simulink library "Ampere_Library"  (R2022b)
settings: Solver=FixedStepDiscrete  StartTime=0  StopTime=10.0  RelTol=1e-3  EnableMultiTasking=on
undefined symbols (not defined in the file or in its folder): A_INST_double, Dem_EventStatusType, ECU_AMBIENT_TEMPERATURE, SET_ECU_AMBIENT_TEMPERATURE, SlDemoSign, Std_ReturnType
libraries: simulink x13
(part 9 of 10)

== system Ampere_Library/User_Defined_Libraries/Timers_and_Counters/A_COUNTER ==
  note: Refer Mask Description of this Library block for detailed information.
  start_flag : Inport  OutDataTypeStr=boolean
      settings: AttributesFormatString=DT = %<OutDataTypeStr>
  ClrVal : Constant  Value=ClrVal  OutDataTypeStr=Inherit: Inherit via back propagation
  IncrVal : Constant  Value=IncrVal  OutDataTypeStr=Inherit: Inherit via back propagation
  Min : MinMax  Inputs=2  InputSameDT=on  RndMeth=Zero
      settings: AttributesFormatString=SAT = %<SaturateOnIntegerOverflow>
  Sum1 : Sum  InputSameDT=on  RndMeth=Zero
      settings: AttributesFormatString=SAT = %<SaturateOnIntegerOverflow>
  Switch1 : Switch  Criteria=u2 ~= 0  Threshold=0.5  RndMeth=Zero  SaturateOnIntegerOverflow=off
      settings: AttributesFormatString=SAT = %<SaturateOnIntegerOverflow>
  UnitDelay : UnitDelay  InitialCondition=IC_zero  SampleTime=-1  HasFrameUpgradeWarning=on
      settings: AttributesFormatString=Init = %<InitialCondition>
  limit_value : Constant  Value=limit_value
  count_value : Outport
  wires:
  start_flag/1 -> Switch1/2
  Sum1/1 -> Min/2
  ClrVal/1 -> Switch1/3
  Switch1/1 -> UnitDelay/1, count_value/1
  IncrVal/1 -> Sum1/2
  Min/1 -> Switch1/1
  limit_value/1 -> Min/1
  UnitDelay/1 -> Sum1/1

== system Ampere_Library/User_Defined_Libraries/Timers_and_Counters/A_Counter_Hold ==
  note: Refer Mask Description of this Library block for detailed information.
  start_flag : Inport  OutDataTypeStr=boolean
      settings: AttributesFormatString=DT = %<OutDataTypeStr>
  clear_flag : Inport  Port=2  OutDataTypeStr=boolean
      settings: AttributesFormatString=DT = %<OutDataTypeStr>
  ClrVal : Constant  Value=ClrVal  OutDataTypeStr=Inherit: Inherit via back propagation
  HoldVal : Constant  Value=HoldVal  OutDataTypeStr=Inherit: Inherit via back propagation
  MinMax : MinMax  Inputs=2  InputSameDT=on  RndMeth=Zero  SaturateOnIntegerOverflow=on
      settings: AttributesFormatString=SAT= %<SaturateOnIntegerOverflow>
  SetVal : Constant  Value=SetVal  OutDataTypeStr=Inherit: Inherit via back propagation
  Sum1 : Sum  InputSameDT=on  RndMeth=Zero  SaturateOnIntegerOverflow=on
      settings: AttributesFormatString=SAT = %<SaturateOnIntegerOverflow>
  Switch : Switch  Criteria=u2 ~= 0  Threshold=0.5  RndMeth=Zero
      settings: AttributesFormatString=SAT = %<SaturateOnIntegerOverflow>
  Switch1 : Switch  Criteria=u2 ~= 0  Threshold=0.5  RndMeth=Zero
      settings: AttributesFormatString=SAT = %<SaturateOnIntegerOverflow>
  UnitDelay : UnitDelay  InitialCondition=count_hold_init  SampleTime=-1  HasFrameUpgradeWarning=on
      settings: AttributesFormatString=Init = %<InitialCondition>\n
  limit_value : Constant  Value=limit_value
  count_value : Outport
  wires:
  SetVal/1 -> Switch/1
  Switch/1 -> Sum1/1
  Sum1/1 -> MinMax/2
  start_flag/1 -> Switch/2
  clear_flag/1 -> Switch1/2
  Switch1/1 -> UnitDelay/1, count_value/1
  HoldVal/1 -> Switch/3
  limit_value/1 -> MinMax/1
  UnitDelay/1 -> Sum1/2
  MinMax/1 -> Switch1/3
  ClrVal/1 -> Switch1/1

== system Ampere_Library/User_Defined_Libraries/Timers_and_Counters/A_IncAndDecCounter ==
  note: Refer Mask Description of this Library block for detailed information.
  Inc_Counter : Inport  OutDataTypeStr=boolean
      settings: AttributesFormatString=DT = %<OutDataTypeStr>
  Dec_Counter : Inport  Port=2  OutDataTypeStr=boolean
      settings: AttributesFormatString=DT = %<OutDataTypeStr>
  Max_Counter : Inport  Port=3
  Min_Counter : Inport  Port=4
  Reset_Counter : Inport  Port=5  OutDataTypeStr=boolean
      settings: AttributesFormatString=DT = %<OutDataTypeStr>
  Counter_Step : Inport  Port=6
  Init_Counter : Inport  Port=7
  Add1 : Sum  InputSameDT=on  RndMeth=Zero
      settings: AttributesFormatString=SAT = %<SaturateOnIntegerOverflow>\n
  Add2 : Sum  Inputs=+-  InputSameDT=on  RndMeth=Zero
      settings: AttributesFormatString=SAT = %<SaturateOnIntegerOverflow>\n
  CONS_ONE : Constant  Value=Cons_One
  CONS_THREE : Constant  Value=Cons_Three
  CONS_TWO : Constant  Value=Cons_Two
  CONS_ZERO : Constant  Value=Cons_Zero
  CONS_ZERO_BP : Constant  Value=Cons_Zero_BP  OutDataTypeStr=Inherit: Inherit via back propagation
  MinMax : MinMax  Inputs=2  InputSameDT=on  RndMeth=Zero
      settings: AttributesFormatString=SAT = %<SaturateOnIntegerOverflow>
  MinMax1 : MinMax  Function=max  Inputs=2  InputSameDT=on  RndMeth=Zero
      settings: AttributesFormatString=SAT = %<SaturateOnIntegerOverflow>
  Multiport_Switch : MultiPortSwitch  DataPortOrder=Zero-based contiguous  DataPortForDefault=Additional data port  DiagnosticForDefault=None  zeroidx=on  RndMeth=Zero  SaturateOnIntegerOverflow=off
      settings: AttributesFormatString=SAT = %<SaturateOnIntegerOverflow>
  Switch{,2..4} (4 alike) : Switch  Criteria=u2 ~= 0  RndMeth=Zero  SaturateOnIntegerOverflow=off
      Switch settings: AttributesFormatString=SAT = %<SaturateOnIntegerOverflow>
  UnitDelay : UnitDelay  InitialCondition=true  SampleTime=-1  HasFrameUpgradeWarning=on
      settings: AttributesFormatString=Init = %<InitialCondition>\n
  Unit_Delay1 : UnitDelay  InitialCondition=false  SampleTime=-1  HasFrameUpgradeWarning=on
      settings: AttributesFormatString=Init = %<InitialCondition>\n
  false : Constant  Value=false
  Counter_Out : Outport
  wires:
  Counter_Step/1 -> Add2/2, Add1/1
  UnitDelay/1 -> Switch/2
  Init_Counter/1 -> Switch/1
  Multiport_Switch/1 -> MinMax/1
  CONS_THREE/1 -> Switch3/3
  MinMax1/1 -> Switch/3
  Min_Counter/1 -> MinMax1/2
  Switch/1 -> Counter_Out/1, Unit_Delay1/1
  CONS_ZERO/1 -> Switch4/1
  MinMax/1 -> MinMax1/1
  Switch2/1 -> Switch4/3
  Unit_Delay1/1 -> Multiport_Switch/5, Add2/1, Add1/2
  Dec_Counter/1 -> Switch2/2
  CONS_ONE/1 -> Switch2/1
  Add2/1 -> Multiport_Switch/3
  Add1/1 -> Multiport_Switch/2
  CONS_TWO/1 -> Switch3/1
  false/1 -> UnitDelay/1
  Switch3/1 -> Switch2/3
  CONS_ZERO_BP/1 -> Multiport_Switch/4
  Switch4/1 -> Multiport_Switch/1
  Max_Counter/1 -> MinMax/2
  Reset_Counter/1 -> Switch3/2
  Inc_Counter/1 -> Switch4/2

== system Ampere_Library/User_Defined_Libraries/Timers_and_Counters/A_Timer_Conversion ==
  note: Refer Mask Description of this Library block for detailed information.
  Timer_To_Adapt : Inport
  Divide : Product  Inputs=*/  RndMeth=Zero
      settings: AttributesFormatString=SAT = %<SaturateOnIntegerOverflow>\n
  RelationalOperator1 : RelationalOperator  Operator=>  OutDataTypeStr=boolean  RndMeth=Zero
  SAMPLE_TIME_CST : Constant  Value=SampleTimeCst  OutDataTypeStr=Inherit: Inherit via back propagation
  Switch : Switch  Criteria=u2 ~= 0  RndMeth=Zero  SaturateOnIntegerOverflow=off
      settings: AttributesFormatString=SAT = %<SaturateOnIntegerOverflow>
  ZERO_CST : Constant  Value=Cons_0  OutDataTypeStr=uint8
      settings: AttributesFormatString=DT = %<OutDataTypeStr>\n
  Timer_Adapted : Outport
  wires:
  Divide/1 -> Switch/1
  Switch/1 -> Timer_Adapted/1
  Timer_To_Adapt/1 -> Divide/1, Switch/3
  RelationalOperator1/1 -> Switch/2
  SAMPLE_TIME_CST/1 -> Divide/2, RelationalOperator1/1
  ZERO_CST/1 -> RelationalOperator1/2

== system Ampere_Library/User_Defined_Libraries/Timers_and_Counters/A_Timer_Dec_Order ==
  note: Detect Increase
  note: Refer Mask Description of this Library block for detailed information.
  Init : Inport
  Duration : Inport  Port=2
  Constant : Constant  Value=Boosting_Factor  OutDataTypeStr=Constant_DT
      settings: AttributesFormatString=DT = %<OutDataTypeStr>\n
  Constant1 : Constant  Value=Boosting_Factor  OutDataTypeStr=Constant_DT
      settings: AttributesFormatString=DT = %<OutDataTypeStr>\n
  Constant2 : Constant  Value=Boosting_Factor  OutDataTypeStr=Constant_DT
      settings: AttributesFormatString=DT = %<OutDataTypeStr>\n
  DataTypeDuplicate : DataTypeDuplicate
  DelayInput1 : UnitDelay  Description=\nStore in Global RAM  InitialCondition=timeoutinit  SampleTime=-1  HasFrameUpgradeWarning=on
      settings: AttributesFormatString=Init = %<InitialCondition>
  DelayInput2 : UnitDelay  Description=\nStore in Global RAM  InitialCondition=Tim1Ini  SampleTime=-1  HasFrameUpgradeWarning=on
      settings: AttributesFormatString=Init = %<InitialCondition>
  DelayInput3 : UnitDelay  Description=\nStore in Global RAM  InitialCondition=initinit  SampleTime=-1  HasFrameUpgradeWarning=on
      settings: AttributesFormatString=Init = %<InitialCondition>
  LogicalOperator : Logic  OutDataTypeStr=boolean
  LogicalOperator1 : Logic  OutDataTypeStr=boolean
  LogicalOperator3 : Logic  Operator=NOT  Inputs=1  OutDataTypeStr=boolean
  Product2 : Product  Inputs=*/  OutDataTypeStr=single  RndMeth=Zero
      settings: AttributesFormatString=DT = %<OutDataTypeStr>\nSAT = %<SaturateOnIntegerOverflow>
  Product3 : Product  OutDataTypeStr=Inherit: Inherit via back propagation  RndMeth=Zero
      settings: AttributesFormatString=SAT = %<SaturateOnIntegerOverflow>
  Product4 : Product  OutDataTypeStr=Inherit: Inherit via back propagation  RndMeth=Zero
      settings: AttributesFormatString=SAT = %<SaturateOnIntegerOverflow>
  RelationalOperator1 : RelationalOperator  Operator=>  OutDataTypeStr=boolean  ZeroCross=off  RndMeth=Zero
  RelationalOperator2 : RelationalOperator  Operator=<=  OutDataTypeStr=boolean  ZeroCross=off  RndMeth=Zero
  Sum : Sum  Inputs=+-  InputSameDT=on  RndMeth=Zero
      settings: AttributesFormatString=SAT = %<SaturateOnIntegerOverflow>
  Switch{1..4} (4 alike) : Switch  Criteria=u2 ~= 0  RndMeth=Zero  SaturateOnIntegerOverflow=off
      Switch2 settings: AttributesFormatString=SAT = %<SaturateOnIntegerOverflow>
      Switch3 settings: AttributesFormatString=SAT = %<SaturateOnIntegerOverflow>
      Switch4 settings: AttributesFormatString=SAT = %<SaturateOnIntegerOverflow>
  TIM1INI3 : Constant  Value=Tim1Ini  OutDataTypeStr=Inherit: Inherit via back propagation
  st : Constant  Value=st  OutDataTypeStr=SampleDT
      settings: AttributesFormatString=DT = %<OutDataTypeStr>\n
  Timeout : Outport
  Timer : Outport  Port=2
  wires:
  Switch3/1 -> Product2/1, DelayInput2/1
  LogicalOperator3/1 -> LogicalOperator1/2
  Duration/1 -> DataTypeDuplicate/2, Product4/1
  Product2/1 -> Timer/1
  Sum/1 -> Switch4/1
  RelationalOperator2/1 -> Switch4/2
  [dly] -> Switch2/1
  Product4/1 -> [dly]
  [Timestep1] -> RelationalOperator1/1
  [Tim1Ini] -> Switch3/1
  DelayInput1/1 -> Switch1/3
  Switch2/1 -> Switch3/3, RelationalOperator1/2
  Init/1 -> LogicalOperator1/1, DelayInput3/1
  Switch1/1 -> LogicalOperator/1, DelayInput1/1
  Product3/1 -> Sum/2, RelationalOperator2/1, [Timestep1]
  Constant1/1 -> Product2/2
  LogicalOperator1/1 -> Switch1/1, Switch1/2, Switch2/2
  LogicalOperator/1 -> Timeout/1
  DelayInput3/1 -> LogicalOperator3/1
  DelayInput2/1 -> RelationalOperator2/2, Sum/1
  Constant/1 -> Product4/2
  st/1 -> Product3/1
  TIM1INI3/1 -> DataTypeDuplicate/1, Switch4/3, [Tim1Ini]
  RelationalOperator1/1 -> Switch3/2, LogicalOperator/2
  Switch4/1 -> Switch2/3
  Constant2/1 -> Product3/2

== system Ampere_Library/User_Defined_Libraries/Timers_and_Counters/A_Timer_Ext_TimeSt ==
  note: Detect Increase
  note: Refer Mask Description of this Library block for detailed information.
  Init : Inport
  Duration : Inport  Port=2
  Timestep : Inport  Port=3
  BOOSTING_FLP : Constant  Value=Boosting_FLP  OutDataTypeStr=Constant_DT
      settings: AttributesFormatString=DT = %<OutDataTypeStr>\n
  BOOSTING_FLP1 : Constant  Value=Boosting_FLP  OutDataTypeStr=Constant_DT
      settings: AttributesFormatString=DT = %<OutDataTypeStr>\n
  BOOSTING_FLP2 : Constant  Value=Boosting_FLP  OutDataTypeStr=Constant_DT
      settings: AttributesFormatString=DT = %<OutDataTypeStr>\n
  DataTypeDuplicate : DataTypeDuplicate  NumInputPorts=3
  DelayInput1 : UnitDelay  Description=\nStore in Global RAM  InitialCondition=timeoutinit  SampleTime=-1  HasFrameUpgradeWarning=on
      settings: AttributesFormatString=Init = %<InitialCondition>\n
  DelayInput2 : UnitDelay  Description=\nStore in Global RAM  InitialCondition=Tim1Ini  SampleTime=-1  HasFrameUpgradeWarning=on
      settings: AttributesFormatString=Init = %<InitialCondition>\n
  DelayInput3 : UnitDelay  Description=\nStore in Global RAM  InitialCondition=initinit  SampleTime=-1  HasFrameUpgradeWarning=on
      settings: AttributesFormatString=Init = %<InitialCondition>\n
  LogicalOperator : Logic  OutDataTypeStr=boolean
  LogicalOperator1 : Logic  OutDataTypeStr=boolean
  LogicalOperator3 : Logic  Operator=NOT  Inputs=1  OutDataTypeStr=boolean
  Product : Product  OutDataTypeStr=Inherit: Inherit via back propagation  RndMeth=Zero
      settings: AttributesFormatString=SAT = %<SaturateOnIntegerOverflow>
  Product1 : Product  OutDataTypeStr=Inherit: Inherit via back propagation  RndMeth=Zero
      settings: AttributesFormatString=SAT = %<SaturateOnIntegerOverflow>
  Product2 : Product  Inputs=*/  OutDataTypeStr=Inherit: Inherit via back propagation  RndMeth=Zero
      settings: AttributesFormatString=SAT = %<SaturateOnIntegerOverflow>
  RelationalOperator1 : RelationalOperator  Operator=>  OutDataTypeStr=boolean  ZeroCross=off  RndMeth=Zero
  RelationalOperator2 : RelationalOperator  Operator=<=  OutDataTypeStr=boolean  ZeroCross=off  RndMeth=Zero
  Sum : Sum  Inputs=+-  InputSameDT=on  RndMeth=Zero
      settings: AttributesFormatString=SAT = %<SaturateOnIntegerOverflow>
  Switch{1..4} (4 alike) : Switch  Criteria=u2 ~= 0  RndMeth=Zero  SaturateOnIntegerOverflow=off
      Switch2 settings: AttributesFormatString=SAT = %<SaturateOnIntegerOverflow>
      Switch3 settings: AttributesFormatString=SAT = %<SaturateOnIntegerOverflow>
      Switch4 settings: AttributesFormatString=SAT = %<SaturateOnIntegerOverflow>
  TIM1INI1 : Constant  Value=Tim1Ini  OutDataTypeStr=Inherit: Inherit via back propagation
  Timeout : Outport
  Timer : Outport  Port=2
  wires:
  DelayInput2/1 -> RelationalOperator2/2, Sum/1
  LogicalOperator1/1 -> Switch1/2, Switch1/1, Switch2/2
  Timestep/1 -> Product/1, DataTypeDuplicate/2
  [Tim1Ini] -> Switch4/3
  [Timestep1] -> RelationalOperator1/1
  [Tim1Ini] -> Switch3/1
  Init/1 -> DelayInput3/1, LogicalOperator1/1
  Switch3/1 -> Product2/1, DelayInput2/1
  LogicalOperator3/1 -> LogicalOperator1/2
  LogicalOperator/1 -> Timeout/1
  Switch1/1 -> DelayInput1/1, LogicalOperator/1
  DelayInput3/1 -> LogicalOperator3/1
  DelayInput1/1 -> Switch1/3
  Switch2/1 -> RelationalOperator1/2, Switch3/3
  Duration/1 -> Product1/1, DataTypeDuplicate/1
  RelationalOperator2/1 -> Switch4/2
  RelationalOperator1/1 -> Switch3/2, LogicalOperator/2
  Switch4/1 -> Switch2/3
  TIM1INI1/1 -> DataTypeDuplicate/3, [Tim1Ini]
  Sum/1 -> Switch4/1
  BOOSTING_FLP1/1 -> Product1/2
  Product2/1 -> Timer/1
  BOOSTING_FLP2/1 -> Product2/2
  Product1/1 -> Switch2/1
  Product/1 -> [Timestep1], RelationalOperator2/1, Sum/2
  BOOSTING_FLP/1 -> Product/2

== system Ampere_Library/User_Defined_Libraries/Timers_and_Counters/A_Timer_Hold_Inc_Order ==
  note: Refer Mask Description of this Library block for detailed information.
  start_flag : Inport
  clear_flag : Inport  Port=2
  target_time : Inport  Port=3
  ClrVal : Constant  Value=ClrVal  OutDataTypeStr=Inherit: Inherit via back propagation
  LogicalOperator2 : Logic  Operator=OR  OutDataTypeStr=boolean
  LogicalOperator3 : Logic  OutDataTypeStr=boolean
  LogicalOperator4 : Logic  Operator=NOT  OutDataTypeStr=boolean
  LogicalOperator5 : Logic  OutDataTypeStr=boolean
  LogicalOperator6 : Logic  Operator=NOT  OutDataTypeStr=boolean
  LogicalOperator7 : Logic  Operator=OR  OutDataTypeStr=boolean
  LogicalOperator8 : Logic  OutDataTypeStr=boolean
  MinMax : MinMax  Inputs=2  InputSameDT=on  RndMeth=Zero
  RelationalOperator : RelationalOperator  Operator=<=  OutDataTypeStr=boolean  RndMeth=Zero
  RelationalOperator1 : RelationalOperator  Operator=<=  OutDataTypeStr=boolean  RndMeth=Zero
  Resol : Constant  Value=Resol  OutDataTypeStr=Inherit: Inherit via back propagation
  Sum : Sum  InputSameDT=on  RndMeth=Zero
  Sum1 : Sum  InputSameDT=on  RndMeth=Zero
  Switch{,1..3} (4 alike) : Switch  Criteria=u2 ~= 0  Threshold=0.5  RndMeth=Zero  SaturateOnIntegerOverflow=off
  TimKill : Constant  Value=TimKill  OutDataTypeStr=Inherit: Inherit via back propagation
  UnitDelay : UnitDelay  InitialCondition=sample_time_init  SampleTime=-1  HasFrameUpgradeWarning=on
      settings: AttributesFormatString=Init = %<InitialCondition>\n
  UnitDelay1 : UnitDelay  InitialCondition=false  SampleTime=-1  HasFrameUpgradeWarning=on
      settings: AttributesFormatString=Init = %<InitialCondition>\n
  UnitDelay2 : UnitDelay  InitialCondition=alarm_init  SampleTime=-1  HasFrameUpgradeWarning=on
      settings: AttributesFormatString=Init = %<InitialCondition>\n
  sample_time : Constant  Value=SampleTime  OutDataTypeStr=Inherit: Inherit via back propagation
  alarm : Outport
  timer_value : Outport  Port=2
  wires:
  LogicalOperator3/1 -> Switch1/1, LogicalOperator5/1, UnitDelay1/1
  Switch1/1 -> alarm/1
  Sum/1 -> Switch/1
  RelationalOperator/1 -> Switch1/3
  LogicalOperator2/1 -> LogicalOperator3/2
  LogicalOperator6/1 -> LogicalOperator3/1, LogicalOperator8/1
  clear_flag/1 -> LogicalOperator7/2, LogicalOperator6/1
  sample_time/1 -> Sum/1
  UnitDelay/1 -> Sum/2, Switch/3
  start_flag/1 -> Switch/2, LogicalOperator8/2
  Switch2/1 -> MinMax/2
  LogicalOperator4/1 -> LogicalOperator5/2
  LogicalOperator8/1 -> LogicalOperator2/1
  LogicalOperator7/1 -> Switch2/2
  UnitDelay1/1 -> LogicalOperator2/2, LogicalOperator4/1
  MinMax/1 -> UnitDelay/1, timer_value/1, Sum1/2
  target_time/1 -> Switch3/1
  TimKill/1 -> RelationalOperator1/2
  Switch3/1 -> RelationalOperator1/1, RelationalOperator/1, UnitDelay2/1, MinMax/1
  ClrVal/1 -> Switch2/1
  RelationalOperator1/1 -> Switch1/2
  Switch/1 -> Switch2/3
  Resol/1 -> Sum1/1
  UnitDelay2/1 -> Switch3/3
  Sum1/1 -> RelationalOperator/2
  LogicalOperator5/1 -> Switch3/2, LogicalOperator7/1

== system Ampere_Library/User_Defined_Libraries/Timers_and_Counters/A_Timer_Inc_Order ==
  note: Detect Increase
  note: Refer Mask Description of this Library block for detailed information.
  start_flag : Inport
  target_time : Inport  Port=2
  ClrVal : Constant  Value=ClrVal  OutDataTypeStr=Inherit: Inherit via back propagation
  LogicalOperator1 : Logic  Operator=NOT  OutDataTypeStr=boolean
  LogicalOperator2 : Logic  OutDataTypeStr=boolean
  LogicalOperator4 : Logic  Operator=NOT  OutDataTypeStr=boolean
  LogicalOperator5 : Logic  OutDataTypeStr=boolean
  LogicalOperator7 : Logic  Operator=OR  OutDataTypeStr=boolean
  MinMax : MinMax  Inputs=2  InputSameDT=on  RndMeth=Zero
  RelationalOperator : RelationalOperator  Operator=<=  OutDataTypeStr=boolean  RndMeth=Zero
  Resol : Constant  Value=Resol  OutDataTypeStr=Inherit: Inherit via back propagation
  Sum : Sum  InputSameDT=on  RndMeth=Zero
  Sum1 : Sum  InputSameDT=on  RndMeth=Zero
  Switch2 : Switch  Criteria=u2 ~= 0  Threshold=0.5  RndMeth=Zero  SaturateOnIntegerOverflow=off
  Switch3 : Switch  Criteria=u2 ~= 0  Threshold=0.5  RndMeth=Zero  SaturateOnIntegerOverflow=off
  UnitDelay : UnitDelay  InitialCondition=Init_val  SampleTime=-1  HasFrameUpgradeWarning=on
      settings: AttributesFormatString=Init = %<InitialCondition>\n
  UnitDelay1 : UnitDelay  InitialCondition=Init_val  SampleTime=-1  HasFrameUpgradeWarning=on
      settings: AttributesFormatString=Init = %<InitialCondition>\n
  UnitDelay2 : UnitDelay  InitialCondition=Init_val  SampleTime=-1  HasFrameUpgradeWarning=on
      settings: AttributesFormatString=Init = %<InitialCondition>\n
  sample_time : Constant  Value=SampleTime  OutDataTypeStr=Inherit: Inherit via back propagation
  alarm : Outport
  timer_value : Outport  Port=2
  wires:
  MinMax/1 -> timer_value/1, Sum1/2, UnitDelay/1
  Switch2/1 -> MinMax/2
  sample_time/1 -> Sum/1
  LogicalOperator7/1 -> Switch2/2
  Resol/1 -> Sum1/1
  LogicalOperator1/1 -> LogicalOperator7/2
  UnitDelay/1 -> Sum/2
  LogicalOperator5/1 -> LogicalOperator7/1, Switch3/2
  target_time/1 -> Switch3/1
  UnitDelay2/1 -> Switch3/3
  RelationalOperator/1 -> LogicalOperator2/2
  Switch3/1 -> MinMax/1, UnitDelay2/1, RelationalOperator/1
  ClrVal/1 -> Switch2/1
  Sum/1 -> Switch2/3
  Sum1/1 -> RelationalOperator/2
  start_flag/1 -> LogicalOperator2/1, LogicalOperator5/1, LogicalOperator1/1, UnitDelay1/1
  LogicalOperator4/1 -> LogicalOperator5/2
  LogicalOperator2/1 -> alarm/1
  UnitDelay1/1 -> LogicalOperator4/1

== system Ampere_Library/User_Defined_Libraries/Timers_and_Counters/A_TurnOffDly_Ctr_Out ==
  note: Refer Mask Description of this Library block for detailed information.
  delay_flag : Inport
  dly : Inport  Port=2
  Boosting_Factor1 : Constant  Value=Boosting_Factor  OutDataTypeStr=Constant_DT
      settings: AttributesFormatString=DT = %<OutDataTypeStr>\n
  Boosting_Factor2 : Constant  Value=Boosting_Factor  OutDataTypeStr=Constant_DT
      settings: AttributesFormatString=DT = %<OutDataTypeStr>\n
  Boosting_Factor3 : Constant  Value=Boosting_Factor  OutDataTypeStr=Constant_DT
      settings: AttributesFormatString=DT = %<OutDataTypeStr>\n
  DataTypeDuplicate : DataTypeDuplicate
  INIVAL2 : Constant  Value=IniVal  OutDataTypeStr=Inherit: Inherit via back propagation
  Logical_Operator1 : Logic  Operator=OR  OutDataTypeStr=boolean
  Product : Product  OutDataTypeStr=Inherit: Inherit via back propagation  RndMeth=Zero
      settings: AttributesFormatString=SAT = %<SaturateOnIntegerOverflow>
  Product1 : Product  OutDataTypeStr=Inherit: Inherit via back propagation  RndMeth=Zero
      settings: AttributesFormatString=SAT = %<SaturateOnIntegerOverflow>
  Product3 : Product  Inputs=*/  OutDataTypeStr=Inherit: Inherit via back propagation  RndMeth=Zero
      settings: AttributesFormatString=SAT = %<SaturateOnIntegerOverflow>\n DT = %<OutDataTypeStr>\n
  Relational_Operator1 : RelationalOperator  Operator=<=  OutDataTypeStr=boolean  RndMeth=Zero
  Relational_Operator8 : RelationalOperator  OutDataTypeStr=boolean  RndMeth=Zero
  Sum1 : Sum  Inputs=+-  InputSameDT=on  OutDataTypeStr=Inherit: Inherit via back propagation  RndMeth=Zero
      settings: AttributesFormatString=SAT = %<SaturateOnIntegerOverflow>
  Switch1 : Switch  Criteria=u2 ~= 0  RndMeth=Zero  SaturateOnIntegerOverflow=off
      settings: AttributesFormatString=SAT = %<SaturateOnIntegerOverflow>
  Switch2 : Switch  Criteria=u2 ~= 0  RndMeth=Zero  SaturateOnIntegerOverflow=off
      settings: AttributesFormatString=SAT = %<SaturateOnIntegerOverflow>
  Switch3 : Switch  Criteria=u2 ~= 0  RndMeth=Zero  SaturateOnIntegerOverflow=off
      settings: AttributesFormatString=SAT = %<SaturateOnIntegerOverflow>
  Ts : Constant  Value=Ts  OutDataTypeStr=SampleDT
      settings: AttributesFormatString=DT = %<OutDataTypeStr>\n
  UnitDelay : UnitDelay  InitialCondition=false  SampleTime=-1  HasFrameUpgradeWarning=on
      settings: AttributesFormatString=Init = %<InitialCondition>
  Unit_Delay2 : UnitDelay  InitialCondition=IniVal  SampleTime=-1  HasFrameUpgradeWarning=on
      settings: AttributesFormatString=Init = %<InitialCondition>
  delay_out : Outport
  ctr : Outport  Port=2
  wires:
  [Timestep] -> Relational_Operator8/2
  Product3/1 -> ctr/1
  Ts/1 -> Product1/1
  Sum1/1 -> Switch3/3
  Switch2/1 -> Switch1/3
  dly/1 -> Product/1, DataTypeDuplicate/2
  Boosting_Factor1/1 -> Product1/2
  [IniVal] -> Switch3/1
  Relational_Operator8/1 -> Logical_Operator1/2
  Boosting_Factor3/1 -> Product/2
  [IniVal] -> Switch1/1
  Logical_Operator1/1 -> delay_out/1
  Boosting_Factor2/1 -> Product3/2
  Product/1 -> Switch2/1
  Unit_Delay2/1 -> Sum1/1, Relational_Operator1/1
  Switch3/1 -> Switch2/3
  Switch1/1 -> Relational_Operator8/1, Product3/1, Unit_Delay2/1
  UnitDelay/1 -> Switch2/2
  delay_flag/1 -> Logical_Operator1/1, Switch1/2, UnitDelay/1
  Product1/1 -> Sum1/2, Relational_Operator1/2, [Timestep]
  Relational_Operator1/1 -> Switch3/2
  INIVAL2/1 -> [IniVal], DataTypeDuplicate/1

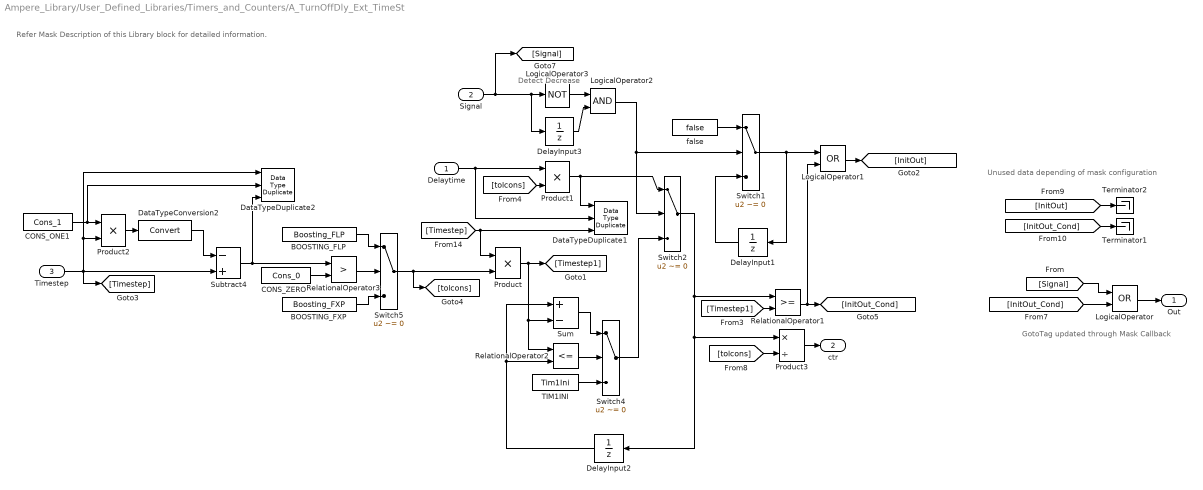
== system Ampere_Library/User_Defined_Libraries/Timers_and_Counters/A_TurnOffDly_Ext_TimeSt ==
  note: Detect Decrease
  note: Unused data depending
      | of mask configuration
  note: GotoTag updated through Mask Callback
  note: Refer Mask Description of this Library block for detailed information.
  Delaytime : Inport
  Signal : Inport  Port=2
  Timestep : Inport  Port=3
  BOOSTING_FLP : Constant  Value=Boosting_FLP  OutDataTypeStr=uint32
      settings: AttributesFormatString=DT = %<OutDataTypeStr>\n
  BOOSTING_FXP : Constant  Value=Boosting_FXP  OutDataTypeStr=Inherit: Inherit via back propagation
  CONS_ONE1 : Constant  Value=Cons_1  OutDataTypeStr=Inherit: Inherit via back propagation
  CONS_ZERO : Constant  Value=Cons_0  OutDataTypeStr=Inherit: Inherit via back propagation
  DataTypeConversion2 : DataTypeConversion  SaturateOnIntegerOverflow=off
      settings: AttributesFormatString=SAT = %<SaturateOnIntegerOverflow>
  DataTypeDuplicate1 : DataTypeDuplicate  NumInputPorts=3
  DataTypeDuplicate2 : DataTypeDuplicate  NumInputPorts=3
  DelayInput1 : UnitDelay  Description=\nStore in Global RAM  InitialCondition=timeoutinit  SampleTime=-1  HasFrameUpgradeWarning=on
      settings: AttributesFormatString=Init = %<InitialCondition>\n
  DelayInput2 : UnitDelay  Description=\nStore in Global RAM  InitialCondition=Tim1Ini  SampleTime=-1  HasFrameUpgradeWarning=on
      settings: AttributesFormatString=Init = %<InitialCondition>\n
  DelayInput3 : UnitDelay  Description=\nStore in Global RAM  InitialCondition=initinit  SampleTime=-1  HasFrameUpgradeWarning=on
      settings: AttributesFormatString=Init = %<InitialCondition>\n
  LogicalOperator : Logic  Operator=OR  OutDataTypeStr=boolean
  LogicalOperator1 : Logic  Operator=OR  OutDataTypeStr=boolean
  LogicalOperator2 : Logic  OutDataTypeStr=boolean
  LogicalOperator3 : Logic  Operator=NOT  Inputs=1  OutDataTypeStr=boolean
  Product : Product  OutDataTypeStr=Inherit: Inherit via back propagation  RndMeth=Zero
      settings: AttributesFormatString=SAT = %<SaturateOnIntegerOverflow>
  Product1 : Product  OutDataTypeStr=Inherit: Inherit via back propagation  RndMeth=Zero
      settings: AttributesFormatString=SAT = %<SaturateOnIntegerOverflow>
  Product2 : Product  OutDataTypeStr=uint32  RndMeth=Zero  SaturateOnIntegerOverflow=on
      settings: AttributesFormatString=SAT = %<SaturateOnIntegerOverflow>\n DT = %<OutDataTypeStr>\n
  Product3 : Product  Inputs=*/  OutDataTypeStr=Inherit: Inherit via back propagation  RndMeth=Zero
      settings: AttributesFormatString=SAT = %<SaturateOnIntegerOverflow>\
  RelationalOperator1 : RelationalOperator  OutDataTypeStr=boolean  ZeroCross=off  RndMeth=Zero
  RelationalOperator2 : RelationalOperator  Operator=<=  OutDataTypeStr=boolean  ZeroCross=off  RndMeth=Zero
  RelationalOperator3 : RelationalOperator  Operator=>  OutDataTypeStr=boolean  ZeroCross=off  RndMeth=Zero
  Subtract4 : Sum  Inputs=-+  InputSameDT=on  OutDataTypeStr=Inherit: Inherit via back propagation  RndMeth=Zero
      settings: AttributesFormatString=SAT = %<SaturateOnIntegerOverflow>
  Sum : Sum  Inputs=+-  InputSameDT=on  OutDataTypeStr=Inherit: Inherit via back propagation  RndMeth=Zero
      settings: AttributesFormatString=SAT = %<SaturateOnIntegerOverflow>
  Switch1 : Switch  Criteria=u2 ~= 0  RndMeth=Zero  SaturateOnIntegerOverflow=off
      settings: AttributesFormatString=SAT = %<SaturateOnIntegerOverflow>
  Switch2 : Switch  Criteria=u2 ~= 0  RndMeth=Zero  SaturateOnIntegerOverflow=off
      settings: AttributesFormatString=SAT = %<SaturateOnIntegerOverflow>
  Switch4 : Switch  Criteria=u2 ~= 0  RndMeth=Zero  SaturateOnIntegerOverflow=off
      settings: AttributesFormatString=SAT = %<SaturateOnIntegerOverflow>
  Switch5 : Switch  Criteria=u2 ~= 0  RndMeth=Zero
      settings: AttributesFormatString=SAT = %<SaturateOnIntegerOverflow>
  TIM1INI : Constant  Value=Tim1Ini  OutDataTypeStr=Inherit: Inherit via back propagation
  Terminator1 : Terminator
  Terminator2 : Terminator
  false : Constant  Value=false
  Out : Outport
  ctr : Outport  Port=2
  wires:
  RelationalOperator1/1 -> LogicalOperator1/2, [InitOut_Cond]
  LogicalOperator2/1 -> Switch1/2, Switch2/2
  [tolcons] -> Product3/2
  RelationalOperator2/1 -> Switch4/2
  [InitOut_Cond] -> LogicalOperator/2
  Subtract4/1 -> DataTypeDuplicate2/3, RelationalOperator3/1
  DelayInput1/1 -> Switch1/3
  Signal/1 -> LogicalOperator3/1, DelayInput3/1, [Signal]
  LogicalOperator/1 -> Out/1
  Switch2/1 -> RelationalOperator1/1, DelayInput2/1, Product3/1
  TIM1INI/1 -> Switch4/3
  Switch5/1 -> Product/2, [tolcons]
  Delaytime/1 -> DataTypeDuplicate1/2, Product1/1
  Product1/1 -> DataTypeDuplicate1/1, Switch2/1
  DataTypeConversion2/1 -> Subtract4/1
  BOOSTING_FLP/1 -> Switch5/1
  CONS_ONE1/1 -> DataTypeDuplicate2/2, Product2/1
  [Timestep1] -> RelationalOperator1/2
  [Timestep] -> DataTypeDuplicate1/3, Product/1
  Product3/1 -> ctr/1
  Switch1/1 -> LogicalOperator1/1, DelayInput1/1
  DelayInput2/1 -> Sum/1, RelationalOperator2/2
  DelayInput3/1 -> LogicalOperator2/2
  [InitOut] -> Terminator2/1
  false/1 -> Switch1/1
  [tolcons] -> Product1/2
  Product/1 -> RelationalOperator2/1, Sum/2, [Timestep1]
  Sum/1 -> Switch4/1
  Switch4/1 -> Switch2/3
  RelationalOperator3/1 -> Switch5/2
  LogicalOperator3/1 -> LogicalOperator2/1
  CONS_ZERO/1 -> RelationalOperator3/2
  Timestep/1 -> DataTypeDuplicate2/1, Product2/2, [Timestep], Subtract4/2
  BOOSTING_FXP/1 -> Switch5/3
  LogicalOperator1/1 -> [InitOut]
  Product2/1 -> DataTypeConversion2/1
  [InitOut_Cond] -> Terminator1/1
  [Signal] -> LogicalOperator/1

== system Ampere_Library/User_Defined_Libraries/Timers_and_Counters/A_TurnOnDly_Ctr_Out ==
  note: Refer Mask Description of this Library block for detailed information.
  delay_flag : Inport
  dly : Inport  Port=2
  Boosting_Factor : Constant  Value=Boosting_Factor  OutDataTypeStr=Constant_DT
      settings: AttributesFormatString=DT = %<OutDataTypeStr>\n
  Boosting_Factor1 : Constant  Value=Boosting_Factor  OutDataTypeStr=Constant_DT
      settings: AttributesFormatString=DT = %<OutDataTypeStr>\n
  Boosting_Factor2 : Constant  Value=Boosting_Factor  OutDataTypeStr=Constant_DT
      settings: AttributesFormatString=DT = %<OutDataTypeStr>\n
  DataTypeDuplicate : DataTypeDuplicate
  INIVAL3 : Constant  Value=IniVal  OutDataTypeStr=Inherit: Inherit via back propagation
  Logical_Operator : Logic  Operator=NOT  OutDataTypeStr=boolean
  Logical_Operator1 : Logic  OutDataTypeStr=boolean
  Logical_Operator6 : Logic  Operator=NOT  OutDataTypeStr=boolean
  Product : Product  OutDataTypeStr=Inherit: Inherit via back propagation  RndMeth=Zero
      settings: AttributesFormatString=SAT = %<SaturateOnIntegerOverflow>
  Product1 : Product  OutDataTypeStr=Inherit: Inherit via back propagation  RndMeth=Zero
      settings: AttributesFormatString=SAT = %<SaturateOnIntegerOverflow>\n
  Product2 : Product  Inputs=*/  OutDataTypeStr=single  RndMeth=Zero
      settings: AttributesFormatString=SAT = %<SaturateOnIntegerOverflow>\n DT = %<OutDataTypeStr>\n
  Relational_Operator1 : RelationalOperator  Operator=<=  OutDataTypeStr=boolean  RndMeth=Zero
  Relational_Operator8 : RelationalOperator  Operator=>  OutDataTypeStr=boolean  RndMeth=Zero
  Sum1 : Sum  Inputs=+-  InputSameDT=on  RndMeth=Zero
      settings: AttributesFormatString=SAT = %<SaturateOnIntegerOverflow>
  Switch1 : Switch  Criteria=u2 ~= 0  RndMeth=Zero  SaturateOnIntegerOverflow=off
  Switch2 : Switch  Criteria=u2 ~= 0  RndMeth=Zero  SaturateOnIntegerOverflow=off
  Switch3 : Switch  Criteria=u2 ~= 0  RndMeth=Zero  SaturateOnIntegerOverflow=off
  Ts : Constant  Value=Ts  OutDataTypeStr=SampleDT
      settings: AttributesFormatString=DT = %<OutDataTypeStr>\n
  UnitDelay : UnitDelay  InitialCondition=false  SampleTime=-1  HasFrameUpgradeWarning=on
      settings: AttributesFormatString=Init = %<InitialCondition>\n
  Unit_Delay2 : UnitDelay  InitialCondition=IniVal  SampleTime=-1  HasFrameUpgradeWarning=on
      settings: AttributesFormatString=Init = %<InitialCondition>\n
  delay_out : Outport
  ctr : Outport  Port=2
  wires:
  Sum1/1 -> Switch3/3
  INIVAL3/1 -> [IniVal], DataTypeDuplicate/1
  Unit_Delay2/1 -> Relational_Operator1/1, Sum1/1
  [IniVal] -> Switch3/1
  [IniVal] -> Switch1/1
  [Timestep] -> Relational_Operator8/1
  Logical_Operator1/1 -> delay_out/1
  Switch2/1 -> Switch1/3
  Ts/1 -> Product/1
  Boosting_Factor/1 -> Product1/2
  delay_flag/1 -> UnitDelay/1, Logical_Operator1/1, Logical_Operator/1
  Switch1/1 -> Unit_Delay2/1, Product2/1, Relational_Operator8/2
  Relational_Operator1/1 -> Switch3/2
  Switch3/1 -> Switch2/3
  Product1/1 -> Switch2/1
  Logical_Operator6/1 -> Switch2/2
  Product2/1 -> ctr/1
  Logical_Operator/1 -> Switch1/2
  Relational_Operator8/1 -> Logical_Operator1/2
  Boosting_Factor1/1 -> Product/2
  Boosting_Factor2/1 -> Product2/2
  Product/1 -> Relational_Operator1/2, Sum1/2, [Timestep]
  UnitDelay/1 -> Logical_Operator6/1
  dly/1 -> DataTypeDuplicate/2, Product1/1

== system Ampere_Library/User_Defined_Libraries/Timers_and_Counters/A_TurnOnDly_Ext_TimeSt ==
  note: Refer Mask Description of this Library block for detailed information.
  Delaytime : Inport
  Signal : Inport  Port=2
  Timestep : Inport  Port=3
  Elab_TimeStepSup : Subsystem
  VariantInitOutput : Subsystem  Variant=on  VariantControlMode=label  LabelModeActiveChoice=(default)
      settings: AttributesFormatString=Active variants=%<CompiledActiveChoiceControl>\n
  Out : Outport
  wires:
  Signal/1 -> VariantInitOutput/1(Signal), Elab_TimeStepSup/1(Signal)
  VariantInitOutput/1(Out) -> Out/1
  Timestep/1 -> Elab_TimeStepSup/2(Timestep)
  Delaytime/1 -> Elab_TimeStepSup/3(Delaytime)
  Elab_TimeStepSup/2(TimeStepSup) -> VariantInitOutput/3(TimeStepSup)
  Elab_TimeStepSup/1(EdgeRising) -> VariantInitOutput/2(EdgeRising)

== system Ampere_Library/MBD_Base_Blocks/Simulink/CommonlyUsedBlocks/Subsystem ==
  note: Subsystem
  In1 : Inport
  Out1 : Outport
  wires:
  In1/1 -> Out1/1

== system Ampere_Library/MBD_Base_Blocks/Simulink/Ports_and_Subsystems/Atomic_Subsystem ==
  note: Atomic_Subsystem
  In1 : Inport
  Out1 : Outport
  wires:
  In1/1 -> Out1/1

== system Ampere_Library/MBD_Base_Blocks/Simulink/Ports_and_Subsystems/CodeReuseSubsystem ==
  note: CodeReuseSubsystem
  In1 : Inport
  Out1 : Outport
  wires:
  In1/1 -> Out1/1

== system Ampere_Library/MBD_Base_Blocks/Simulink/Ports_and_Subsystems/Enabled_Subsystem ==
  note: Enabled_Subsystem
  In1 : Inport
  Enable : EnablePort
      settings: AttributesFormatString=%<StatesWhenEnabling>\n
  Out1 : Outport
      settings: AttributesFormatString=Init = %<InitialOutput>
  wires:
  In1/1 -> Out1/1

== system Ampere_Library/MBD_Base_Blocks/Simulink/Ports_and_Subsystems/Enabled_and_Triggered_Subsystem ==
  note: Enabled_and_Triggered_Subsystem
  In1 : Inport
  Enable : EnablePort
      settings: AttributesFormatString=%<StatesWhenEnabling>\n
  Trigger : TriggerPort  VariantControl=Variant  SampleTime=-1
  Out1 : Outport
      settings: AttributesFormatString=Init = %<InitialOutput>
  wires:
  In1/1 -> Out1/1

== system Ampere_Library/MBD_Base_Blocks/Simulink/Ports_and_Subsystems/ForEachSubsystem ==
  note: ForEach_Subsystem
  In1 : Inport  Partition=on  PartitionDimension=1  PartitionWidth=1  PartitionOffset=0
  ForEach : ForEach  DisableCoverage=on
  Out1 : Outport  ConcatenationDimension=1
  wires:
  In1/1 -> Out1/1

== system Ampere_Library/MBD_Base_Blocks/Simulink/Ports_and_Subsystems/For_Iterator_Subsystem ==
  note: For_Iterator_Subsystem
  In1 : Inport
  For_Iterator : ForIterator  IndexMode=Zero-based
      settings: AttributesFormatString=|
      | N = %<IterationLimit>
      | %<ResetStates>\n
  Out1 : Outport
  wires:
  In1/1 -> Out1/1

== system Ampere_Library/MBD_Base_Blocks/Simulink/Ports_and_Subsystems/Function_Call_Subsystem ==
  note: Function_Call_Subsystem
  In1 : Inport
  function : TriggerPort  TriggerType=function-call  VariantControl=Variant  SampleTime=-1
      settings: AttributesFormatString=%<StatesWhenEnabling>
  Out1 : Outport
  wires:
  In1/1 -> Out1/1

== system Ampere_Library/MBD_Base_Blocks/Simulink/Ports_and_Subsystems/If_Action_Subsystem ==
  note: If_Action_Subsystem
  In1 : Inport
  Action_Port : ActionPort
  Out1 : Outport
  wires:
  In1/1 -> Out1/1

== system Ampere_Library/MBD_Base_Blocks/Simulink/Ports_and_Subsystems/Model_Variants ==
  note: Model Variants
  <Enter Model Name> : ModelReference  SimulationMode=Normal  VariantControl=Variant1
      settings: AttributesFormatString=Active variants=%<ActiveVariant>\n
  <Enter Model Name>1 : ModelReference  SimulationMode=Normal  VariantControl=Variant2
      settings: AttributesFormatString=Active variants=%<ActiveVariant>\n

== system Ampere_Library/MBD_Base_Blocks/Simulink/Ports_and_Subsystems/Subsystem ==
  note: Subsystem
  In1 : Inport
  Out1 : Outport
  wires:
  In1/1 -> Out1/1

== system Ampere_Library/MBD_Base_Blocks/Simulink/Ports_and_Subsystems/Switch_Case_Action_Subsystem ==
  note: Switch_Case_Action_Subsystem
  In1 : Inport
  Action_Port : ActionPort
  Out1 : Outport
  wires:
  In1/1 -> Out1/1

== system Ampere_Library/MBD_Base_Blocks/Simulink/Ports_and_Subsystems/Triggered_Subsystem ==
  note: Triggered_Subsystem
  In1 : Inport
  Trigger : TriggerPort  VariantControl=Variant  SampleTime=-1
  Out1 : Outport
      settings: AttributesFormatString=Init = %<InitialOutput>
  wires:
  In1/1 -> Out1/1

== system Ampere_Library/MBD_Base_Blocks/Simulink/Ports_and_Subsystems/Variant_subsystem ==
  note: 1) Only subsystems can be added as variant choices at this level
      | 2) Blocks cannot be connected at this level as connectivity is
      | automatically determined at simulation, based on the active variant
  In1 : Inport
  Out1 : Outport

== system Ampere_Library/MBD_Base_Blocks/Simulink/Ports_and_Subsystems/While_Iterator_Subsystem ==
  note: While_Iterator_Subsystem
  In1 : Inport
  While_Iterator : WhileIterator
      settings: AttributesFormatString=|
      | Max iteration = %<MaxIters>
      | %<ResetStates>\n
  Out1 : Outport
      settings: AttributesFormatString=Init = %<InitialOutput>
  wires:
  In1/1 -> Out1/1

== system Ampere_Library/MBD_Base_Blocks/Simulink/User_Defined_Functions/Initialize_Function ==
  note: Initialize Function
  Constant : Constant  DisableCoverage=on  Value=false
  Event_Listener : EventListener  EventName=reset
  Out1 : Outport
  wires:
  Constant/1 -> Out1/1

== system Ampere_Library/MBD_Base_Blocks/Simulink/User_Defined_Functions/Simulink_Function ==
  note: Simulink Function
  f : TriggerPort  TriggerType=function-call  IsSimulinkFunction=on  FunctionName=f  FunctionVisibility=scoped  VariantControl=(inherit)
  u : ArgIn  DisableCoverage=on  ArgumentName=u
  y : ArgOut  DisableCoverage=on  ArgumentName=y
  wires:
  u/1 -> y/1

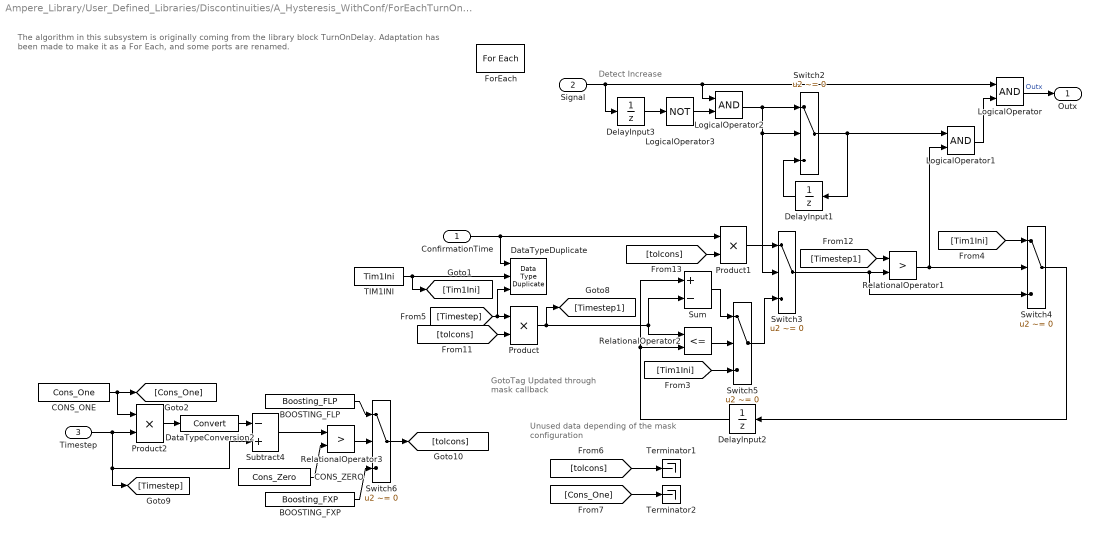
== system Ampere_Library/User_Defined_Libraries/Discontinuities/A_Hysteresis_WithConf/ForEachTurnOnDelay ==
  note: Detect Increase
  note: GotoTag Updated
      | through mask callback
  note: Unused data depending
      | of the mask configuration
  note: The algorithm in this subsystem is originally coming from the library block TurnOnDelay.
      | Adaptation has been made to make it as a For Each, and some ports are renamed.
  ConfirmationTime : Inport
  Signal : Inport  Port=2  Partition=on  PartitionDimension=1  PartitionWidth=1  PartitionOffset=0
  Timestep : Inport  Port=3
  BOOSTING_FLP : Constant  Value=Boosting_FLP  OutDataTypeStr=uint32
      settings: AttributesFormatString=DT = %<OutDataTypeStr>\n
  BOOSTING_FXP : Constant  Value=Boosting_FXP  OutDataTypeStr=Inherit: Inherit via back propagation
  CONS_ONE : Constant  Value=Cons_One  OutDataTypeStr=Inherit: Inherit via back propagation
  CONS_ZERO : Constant  Value=Cons_Zero  OutDataTypeStr=Inherit: Inherit via back propagation
  DataTypeConversion2 : DataTypeConversion  SaturateOnIntegerOverflow=off
      settings: AttributesFormatString=SAT = %<SaturateOnIntegerOverflow>
  DataTypeDuplicate : DataTypeDuplicate  NumInputPorts=3
  DelayInput1 : UnitDelay  Description=\nStore in Global RAM  InitialCondition=timeoutinit  SampleTime=-1  HasFrameUpgradeWarning=on
      settings: AttributesFormatString=Init = %<InitialCondition>
  DelayInput2 : UnitDelay  Description=\nStore in Global RAM  InitialCondition=Tim1Ini  SampleTime=-1  HasFrameUpgradeWarning=on
      settings: AttributesFormatString=Init = %<InitialCondition>
  DelayInput3 : UnitDelay  Description=\nStore in Global RAM  InitialCondition=initinit  SampleTime=-1  HasFrameUpgradeWarning=on
      settings: AttributesFormatString=Init = %<InitialCondition>
  ForEach : ForEach  DisableCoverage=on
  LogicalOperator : Logic  OutDataTypeStr=boolean
  LogicalOperator1 : Logic  OutDataTypeStr=boolean
  LogicalOperator2 : Logic  OutDataTypeStr=boolean
  LogicalOperator3 : Logic  Operator=NOT  Inputs=1  OutDataTypeStr=boolean
  Product : Product  OutDataTypeStr=Inherit: Inherit via back propagation  RndMeth=Zero
      settings: AttributesFormatString=SAT = %<SaturateOnIntegerOverflow>
  Product1 : Product  OutDataTypeStr=Inherit: Inherit via back propagation  RndMeth=Zero
      settings: AttributesFormatString=SAT = %<SaturateOnIntegerOverflow>
  Product2 : Product  InputSameDT=on  OutDataTypeStr=uint32  RndMeth=Zero  SaturateOnIntegerOverflow=on
      settings: AttributesFormatString=|
      | DT = %<OutDataTypeStr>
      | SAT = %<SaturateOnIntegerOverflow>
  RelationalOperator1 : RelationalOperator  Operator=>  OutDataTypeStr=boolean  ZeroCross=off  RndMeth=Zero
  RelationalOperator2 : RelationalOperator  Operator=<=  OutDataTypeStr=boolean  ZeroCross=off  RndMeth=Zero
  RelationalOperator3 : RelationalOperator  Operator=>  OutDataTypeStr=boolean  ZeroCross=off  RndMeth=Zero
  Subtract4 : Sum  Inputs=-+  InputSameDT=on  RndMeth=Zero
      settings: AttributesFormatString=SAT = %<SaturateOnIntegerOverflow>
  Sum : Sum  Inputs=+-  InputSameDT=on  OutDataTypeStr=Inherit: Inherit via back propagation  RndMeth=Zero
      settings: AttributesFormatString=SAT = %<SaturateOnIntegerOverflow>
  Switch{2..5} (4 alike) : Switch  Criteria=u2 ~= 0  RndMeth=Zero  SaturateOnIntegerOverflow=off
      Switch3 settings: AttributesFormatString=SAT = %<SaturateOnIntegerOverflow>
      Switch4 settings: AttributesFormatString=SAT = %<SaturateOnIntegerOverflow>
      Switch5 settings: AttributesFormatString=SAT = %<SaturateOnIntegerOverflow>
  Switch6 : Switch  Criteria=u2 ~= 0  RndMeth=Zero
      settings: AttributesFormatString=SAT = %<SaturateOnIntegerOverflow>
  TIM1INI : Constant  Value=Tim1Ini  OutDataTypeStr=Inherit: Inherit via back propagation
  Terminator1 : Terminator
  Terminator2 : Terminator
  Outx : Outport  ConcatenationDimension=1
  wires:
  [Timestep] -> DataTypeDuplicate/3, Product/1
  Timestep/1 -> [Timestep], Subtract4/2, Product2/2
  RelationalOperator3/1 -> Switch6/2
  BOOSTING_FLP/1 -> Switch6/1
  LogicalOperator2/1 -> Switch2/2, Switch3/2, Switch2/1
  [Timestep1] -> RelationalOperator1/1
  [Tim1Ini] -> Switch5/3
  Product/1 -> [Timestep1], Sum/2, RelationalOperator2/1
  LogicalOperator/1 -> Outx/1  "Outx"
  [Tim1Ini] -> Switch4/1
  Sum/1 -> Switch5/1
  Switch2/1 -> LogicalOperator1/1, DelayInput1/1
  Switch6/1 -> [tolcons]
  RelationalOperator2/1 -> Switch5/2
  LogicalOperator1/1 -> LogicalOperator/2
  Switch4/1 -> DelayInput2/1
  DelayInput2/1 -> Sum/1, RelationalOperator2/2
  [tolcons] -> Terminator1/1
  Product2/1 -> DataTypeConversion2/1
  Product1/1 -> Switch3/1
  DelayInput1/1 -> Switch2/3
  LogicalOperator3/1 -> LogicalOperator2/2
  Switch5/1 -> Switch3/3
  RelationalOperator1/1 -> LogicalOperator1/2, Switch4/2
  Switch3/1 -> Switch4/3, RelationalOperator1/2
  [tolcons] -> Product1/2
  ConfirmationTime/1 -> DataTypeDuplicate/1, Product1/1
  DataTypeConversion2/1 -> Subtract4/1
  [tolcons] -> Product/2
  CONS_ONE/1 -> [Cons_One], Product2/1
  CONS_ZERO/1 -> RelationalOperator3/2
  Signal/1 -> DelayInput3/1, LogicalOperator2/1, LogicalOperator/1
  [Cons_One] -> Terminator2/1
  Subtract4/1 -> RelationalOperator3/1
  BOOSTING_FXP/1 -> Switch6/3
  TIM1INI/1 -> [Tim1Ini], DataTypeDuplicate/2
  DelayInput3/1 -> LogicalOperator3/1
